simulink model "Tiny_M23"  (R2017b)
settings: Solver=VariableStepAuto  StartTime=0.0  StopTime=10.0  RelTol=1e-3
settings Model: Creator=ainhoa.arruabarrena  LastModifiedBy=ainhoa.arruabarrena

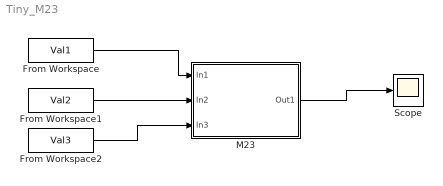
== system Tiny_M23 ==
  From Workspace : FromWorkspace  VariableName=Val1  SampleTime=0
  From Workspace1 : FromWorkspace  VariableName=Val2  SampleTime=0
  From Workspace2 : FromWorkspace  VariableName=Val3  SampleTime=0
  M23 : Subsystem
  Scope : Scope
  wires:
  From Workspace2/1 -> M23/3(In3)
  From Workspace1/1 -> M23/2(In2)
  From Workspace/1 -> M23/1(In1)
  M23/1(Out1) -> Scope/1

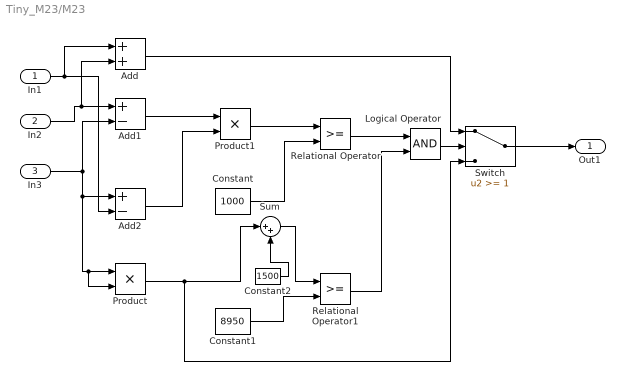
== system Tiny_M23/M23 ==
  In1 : Inport
  In2 : Inport  Port=2
  In3 : Inport  Port=3
  Add : Sum
  Add1 : Sum  Inputs=+-
  Add2 : Sum  Inputs=+-
  Constant : Constant  Value=1000
  Constant1 : Constant  Value=8950
  Constant2 : Constant  Value=1500
  Logical Operator : Logic  AllPortsSameDT=off  OutDataTypeStr=boolean
  Product : Product
  Product1 : Product
  Relational Operator : RelationalOperator  OutDataTypeStr=boolean  RndMeth=Nearest
  Relational Operator1 : RelationalOperator  OutDataTypeStr=boolean  RndMeth=Nearest
  Sum : Sum  Inputs=|++
  Switch : Switch  Threshold=1
  Out1 : Outport
  wires:
  In3/1 -> Add2/1, Product/2, Product/1, Add1/2
  In1/1 -> Add/1, Add2/2
  In2/1 -> Add/2, Add1/1
  Add1/1 -> Product1/1
  Add2/1 -> Product1/2
  Product1/1 -> Relational Operator/1
  Product/1 -> Sum/1, Switch/3
  Constant/1 -> Relational Operator/2
  Constant1/1 -> Relational Operator1/2
  Relational Operator/1 -> Logical Operator/1
  Relational Operator1/1 -> Logical Operator/2
  Logical Operator/1 -> Switch/2
  Add/1 -> Switch/1
  Switch/1 -> Out1/1
  Sum/1 -> Relational Operator1/1
  Constant2/1 -> Sum/2
